simulink model "motor_uart"  (R2024b)
settings: Solver=FixedStepDiscrete  StartTime=0.0  StopTime=inf  FixedStep=0.01  RelTol=1e-3
undefined symbols (not defined in the file): LF
libraries: instrumentseriallib x3
settings Model: Creator=USER  LastModifiedBy=USER

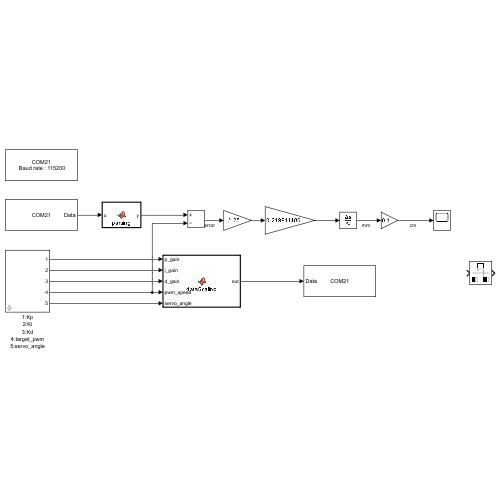
[thumbnail: Simulink's stored preview of the top-level diagram]
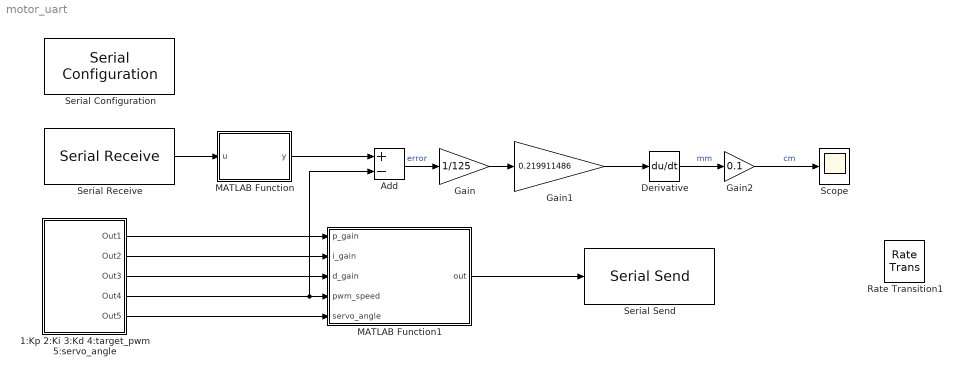
== system motor_uart ==
  1:Kp 2:Ki 3:Kd 4:target_pwm 5:servo_angle : Subsystem  mask{P_gain=1.55, I_gain=2.65, D_gain=0.001, PWM_speed=0, Servo_angle=0}
      mask prompts: P_gain "P gain"; I_gain "I gain"; D_gain "D gain"; PWM_speed "PWM Speed"; Servo_angle "Servo Angle"
      mask DialogControl ParameterGroupVar Prompt: 파라미터
  Add : Sum  Inputs=+-
  Derivative : Derivative
  Gain : Gain  Gain=1/125
  Gain1 : Gain  Gain=0.219911486
  Gain2 : Gain  Gain=0.1
  MATLAB Function : MATLAB Function  TreatAsAtomicUnit=on
  MATLAB Function1 : MATLAB Function  TreatAsAtomicUnit=on
  Rate Transition1 : RateTransition  Integrity=off  OutPortSampleTime=0.5
  Scope : Scope
  Serial Configuration : instrumentseriallib/Serial Configuration  Priority=-200000  PortSel=COM21  Port=COM21  ComPort=COM21  BaudRate=115200  DataBits=8  Parity=none  StopBits=1  ByteOrder=big-endian  FlowControl=none  Timeout=1  SimulateUsing=Interpreted execution  BlockInModel=on  aMode=1
  Serial Receive : instrumentseriallib/Serial Receive  Priority=1  PortSel=COM21  Port=COM21  ComPort=COM21  DataType=uint8  SaveDataType=uint8  ToggleHeader=off  Header=[]  ToggleDataSize=on  DataSize=[1 5]  ToggleTerminator=on  Terminator=LF ('\n')  CustomTerminator=[]  InputFormat=Column major  EnableBlockingMode=on  ActionDataUnavailable=Output last received value  ActionWhenDataUnavailable=Output last received value  CustomValue=0  SampleTime=0.01  SimulateUsing=Interpreted execution  BlockInModel=on  aMode=1
  Serial Send : instrumentseriallib/Serial Send  Priority=1  PortSel=COM21  Port=COM21  ComPort=COM21  Header=[]  Terminator=<none>  CustomTerminator=[]  EnableBlockingMode=on  SimulateUsing=Interpreted execution  BlockInModel=on  aMode=1
  wires:
  Serial Receive/1 -> MATLAB Function/1(u)
  1:Kp 2:Ki 3:Kd 4:target_pwm 5:servo_angle/4(Out4) -> Add/2, MATLAB Function1/4(pwm_speed)
  1:Kp 2:Ki 3:Kd 4:target_pwm 5:servo_angle/1(Out1) -> MATLAB Function1/1(p_gain)
  1:Kp 2:Ki 3:Kd 4:target_pwm 5:servo_angle/2(Out2) -> MATLAB Function1/2(i_gain)
  1:Kp 2:Ki 3:Kd 4:target_pwm 5:servo_angle/3(Out3) -> MATLAB Function1/3(d_gain)
  MATLAB Function1/1(out) -> Serial Send/1
  1:Kp 2:Ki 3:Kd 4:target_pwm 5:servo_angle/5(Out5) -> MATLAB Function1/5(servo_angle)
  MATLAB Function/1(y) -> Add/1
  Add/1 -> Gain/1  "error"
  Gain/1 -> Gain1/1
  Gain1/1 -> Derivative/1
  Derivative/1 -> Gain2/1  "mm"
  Gain2/1 -> Scope/1  "cm"

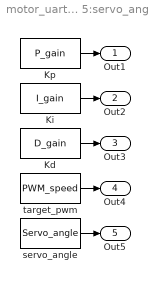
== system motor_uart/1:Kp 2:Ki 3:Kd 4:target_pwm 5:servo_angle ==
  Kd : Constant  Value=D_gain
  Ki : Constant  Value=I_gain
  Kp : Constant  Value=P_gain
  servo_angle : Constant  Value=Servo_angle
  target_pwm : Constant  Value=PWM_speed
  Out1 : Outport
  Out2 : Outport  Port=2
  Out3 : Outport  Port=3
  Out4 : Outport  Port=4
  Out5 : Outport  Port=5
  wires:
  Kd/1 -> Out3/1
  Kp/1 -> Out1/1
  Ki/1 -> Out2/1
  target_pwm/1 -> Out4/1
  servo_angle/1 -> Out5/1

== matlab function motor_uart/MATLAB Function1 ==
  data: p_gain input; out output; i_gain input; d_gain input; pwm_speed input; servo_angle input
function out = dataScaling(p_gain, i_gain, d_gain, pwm_speed, servo_angle)
    % 데이터 스케일링
    p_uint16 = uint16(p_gain * 1000);
    i_uint16 = uint16(i_gain * 1000);
    d_uint16 = uint16(d_gain * 1000);
    pwm_uint16 = uint16(pwm_speed + 5000);
    servo_uint8 = uint8(servo_angle + 50);

    % 각 uint16 값을 상위/하위 바이트로 분리
    p_high = uint8(bitshift(p_uint16, -8));
    p_low = uint8(bitand(p_uint16, 255));
    
    i_high = uint8(bitshift(i_uint16, -8));
    i_low = uint8(bitand(i_uint16, 255));
    
    d_high = uint8(bitshift(d_uint16, -8));
    d_low = uint8(bitand(d_uint16, 255));
    
    pwm_high = uint8(bitshift(pwm_uint16, -8));
    pwm_low = uint8(bitand(pwm_uint16, 255));
    
    % 전송할 순서대로 바이트 배열 구성
    out = [p_high; p_low; i_high; i_low; d_high; d_low; pwm_high; pwm_low; servo_uint8;];
end

== matlab function motor_uart/MATLAB Function ==
  data: u input; y output
function y = parsing(u)
    u_double = double(u);

    digits = u_double - 48;
    n = length(digits);

    data = 0;
    for a=0:(n - 2)
        data = data + digits(n - a - 1) * power(10, a);
    end

    if (digits(5) == (uint8('m') - 48))
        data = -data;
    end


    y = data;
end
